simulink model "hnn_3_neurons"  (R2024b)
settings: Solver=VariableStepAuto  StartTime=0.0  StopTime=10.0  RelTol=1e-3
settings Model: Creator=merlin  LastModifiedBy=merlin

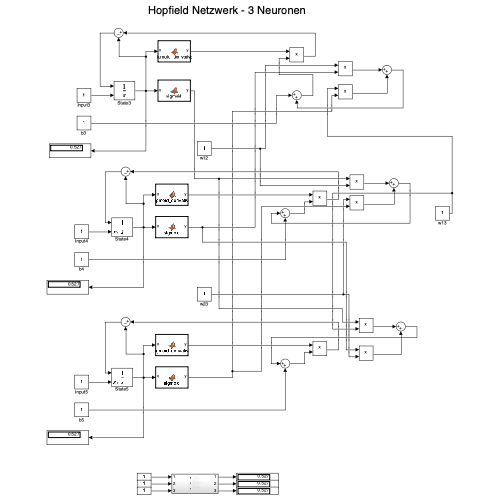
[thumbnail: Simulink's stored preview of the top-level diagram]
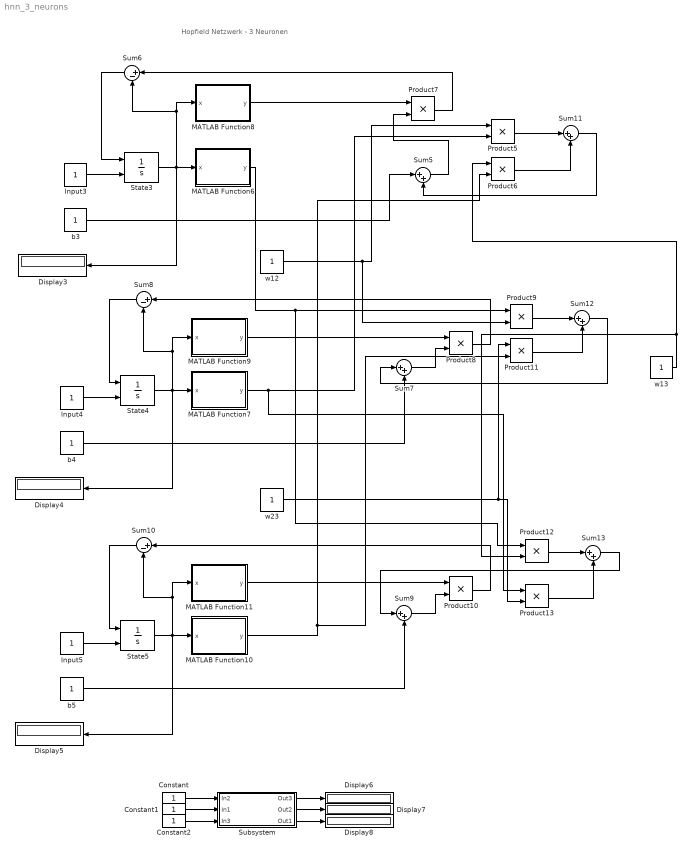
== system hnn_3_neurons ==
  note: Hopfield Netzwerk - 3 Neuronen
  Constant : Constant
  Constant1 : Constant
  Constant2 : Constant
  Display{3..8} (6 alike) : Display
  Input3 : Constant
  Input4 : Constant
  Input5 : Constant
  MATLAB Function10 : MATLAB Function  TreatAsAtomicUnit=on
  MATLAB Function11 : MATLAB Function  TreatAsAtomicUnit=on
  MATLAB Function6 : MATLAB Function  TreatAsAtomicUnit=on
  MATLAB Function7 : MATLAB Function  TreatAsAtomicUnit=on
  MATLAB Function8 : MATLAB Function  TreatAsAtomicUnit=on
  MATLAB Function9 : MATLAB Function  TreatAsAtomicUnit=on
  Product{5..13} (9 alike) : Product
  State3 : Integrator  InitialConditionSource=external
  State4 : Integrator  InitialConditionSource=external
  State5 : Integrator  InitialConditionSource=external
  Subsystem : Subsystem
  Sum10 : Sum  Inputs=|+-
  Sum{5,7,9,11..13} (6 alike) : Sum  Inputs=|++
  Sum6 : Sum  Inputs=|+-
  Sum8 : Sum  Inputs=|+-
  b3 : Constant
  b4 : Constant
  b5 : Constant
  w12 : Constant
  w13 : Constant
  w23 : Constant
  wires:
  w12/1 -> Product9/2, Product5/1
  MATLAB Function7/1(y) -> Product13/1, Product5/2
  Product8/1 -> Sum8/1
  State5/1 -> Display5/1, Sum10/2, MATLAB Function11/1(x), MATLAB Function10/1(x)
  Subsystem/3(Out1) -> Display8/1
  Product7/1 -> Sum6/1
  b3/1 -> Sum5/1
  Input3/1 -> State3/2
  Sum13/1 -> Sum9/1
  Product10/1 -> Sum10/1
  Product13/1 -> Sum13/2
  Subsystem/1(Out3) -> Display6/1
  Sum11/1 -> Sum5/2
  Product6/1 -> Sum11/2
  Input4/1 -> State4/2
  Sum6/1 -> State3/1
  Sum9/1 -> Product10/2
  Sum10/1 -> State5/1
  MATLAB Function8/1(y) -> Product7/1
  w13/1 -> Product12/2, Product6/1
  State4/1 -> Display4/1, Sum8/2, MATLAB Function9/1(x), MATLAB Function7/1(x)
  Constant2/1 -> Subsystem/3(In3)
  b5/1 -> Sum9/2
  Product9/1 -> Sum12/1
  MATLAB Function11/1(y) -> Product10/1
  Subsystem/2(Out2) -> Display7/1
  Sum5/1 -> Product7/2
  Product11/1 -> Sum12/2
  Sum12/1 -> Sum7/1
  Input5/1 -> State5/2
  Product5/1 -> Sum11/1
  Product12/1 -> Sum13/1
  Constant1/1 -> Subsystem/2(In1)
  MATLAB Function10/1(y) -> Product11/2, Product6/2
  b4/1 -> Sum7/2
  State3/1 -> Display3/1, Sum6/2, MATLAB Function8/1(x), MATLAB Function6/1(x)
  MATLAB Function9/1(y) -> Product8/1
  Sum8/1 -> State4/1
  Sum7/1 -> Product8/2
  MATLAB Function6/1(y) -> Product12/1, Product9/1
  Constant/1 -> Subsystem/1(In2)
  w23/1 -> Product13/2, Product11/1

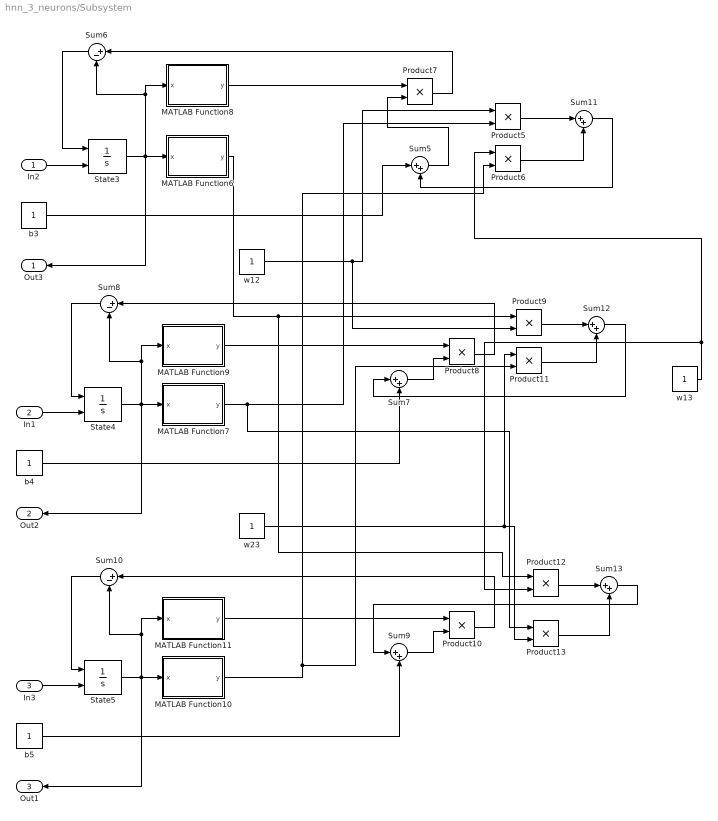
== system hnn_3_neurons/Subsystem ==
  In2 : Inport
  In1 : Inport  Port=2
  In3 : Inport  Port=3
  MATLAB Function10 : MATLAB Function  TreatAsAtomicUnit=on
  MATLAB Function11 : MATLAB Function  TreatAsAtomicUnit=on
  MATLAB Function6 : MATLAB Function  TreatAsAtomicUnit=on
  MATLAB Function7 : MATLAB Function  TreatAsAtomicUnit=on
  MATLAB Function8 : MATLAB Function  TreatAsAtomicUnit=on
  MATLAB Function9 : MATLAB Function  TreatAsAtomicUnit=on
  Product{5..13} (9 alike) : Product
  State3 : Integrator  InitialConditionSource=external
  State4 : Integrator  InitialConditionSource=external
  State5 : Integrator  InitialConditionSource=external
  Sum10 : Sum  Inputs=|+-
  Sum{5,7,9,11..13} (6 alike) : Sum  Inputs=|++
  Sum6 : Sum  Inputs=|+-
  Sum8 : Sum  Inputs=|+-
  b3 : Constant
  b4 : Constant
  b5 : Constant
  w12 : Constant
  w13 : Constant
  w23 : Constant
  Out3 : Outport
  Out2 : Outport  Port=2
  Out1 : Outport  Port=3
  wires:
  Product9/1 -> Sum12/1
  b5/1 -> Sum9/2
  Product13/1 -> Sum13/2
  Sum5/1 -> Product7/2
  b4/1 -> Sum7/2
  Sum10/1 -> State5/1
  MATLAB Function7/1(y) -> Product13/1, Product5/2
  MATLAB Function9/1(y) -> Product8/1
  Product5/1 -> Sum11/1
  w12/1 -> Product9/2, Product5/1
  Sum13/1 -> Sum9/1
  State5/1 -> Out1/1, Sum10/2, MATLAB Function11/1(x), MATLAB Function10/1(x)
  MATLAB Function8/1(y) -> Product7/1
  MATLAB Function11/1(y) -> Product10/1
  Sum9/1 -> Product10/2
  MATLAB Function6/1(y) -> Product12/1, Product9/1
  Product12/1 -> Sum13/1
  MATLAB Function10/1(y) -> Product11/2, Product6/2
  State4/1 -> Out2/1, Sum8/2, MATLAB Function9/1(x), MATLAB Function7/1(x)
  Sum8/1 -> State4/1
  Product8/1 -> Sum8/1
  State3/1 -> Out3/1, Sum6/2, MATLAB Function8/1(x), MATLAB Function6/1(x)
  Sum6/1 -> State3/1
  Product7/1 -> Sum6/1
  b3/1 -> Sum5/1
  Product6/1 -> Sum11/2
  In1/1 -> State4/2
  Sum7/1 -> Product8/2
  In3/1 -> State5/2
  w23/1 -> Product13/2, Product11/1
  Product11/1 -> Sum12/2
  Sum12/1 -> Sum7/1
  Sum11/1 -> Sum5/2
  Product10/1 -> Sum10/1
  w13/1 -> Product12/2, Product6/1
  In2/1 -> State3/2

== matlab function hnn_3_neurons/MATLAB Function7 ==
  data: x input; y output
function y = sigmoid(x)
y = 1 ./ (1 + exp(-x));
end

== matlab function hnn_3_neurons/MATLAB Function8 ==
  data: x input; y output
function y = sigmoid_derivative(x)
sigmoid = 1 ./ (1 + exp(-x));
y = sigmoid .* (1 - sigmoid);
end

== matlab function hnn_3_neurons/MATLAB Function9 ==
  data: x input; y output
function y = sigmoid_derivative(x)
sigmoid = 1 ./ (1 + exp(-x));
y = sigmoid .* (1 - sigmoid);
end

== matlab function hnn_3_neurons/MATLAB Function10 ==
  data: x input; y output
function y = sigmoid(x)
y = 1 ./ (1 + exp(-x));
end

== matlab function hnn_3_neurons/MATLAB Function11 ==
  data: x input; y output
function y = sigmoid_derivative(x)
sigmoid = 1 ./ (1 + exp(-x));
y = sigmoid .* (1 - sigmoid);
end

== matlab function hnn_3_neurons/Subsystem/MATLAB Function10 ==
  data: x input; y output
function y = sigmoid(x)
y = 1 ./ (1 + exp(-x));
end

== matlab function hnn_3_neurons/Subsystem/MATLAB Function11 ==
  data: x input; y output
function y = sigmoid_derivative(x)
sigmoid = 1 ./ (1 + exp(-x));
y = sigmoid .* (1 - sigmoid);
end

== matlab function hnn_3_neurons/Subsystem/MATLAB Function6 ==
  data: x input; y output
function y = sigmoid(x)
y = 1 ./ (1 + exp(-x));
end

== matlab function hnn_3_neurons/MATLAB Function6 ==
  data: x input; y output
function y = sigmoid(x)
y = 1 ./ (1 + exp(-x));
end

== matlab function hnn_3_neurons/Subsystem/MATLAB Function7 ==
  data: x input; y output
function y = sigmoid(x)
y = 1 ./ (1 + exp(-x));
end

== matlab function hnn_3_neurons/Subsystem/MATLAB Function8 ==
  data: x input; y output
function y = sigmoid_derivative(x)
sigmoid = 1 ./ (1 + exp(-x));
y = sigmoid .* (1 - sigmoid);
end

== matlab function hnn_3_neurons/Subsystem/MATLAB Function9 ==
  data: x input; y output
function y = sigmoid_derivative(x)
sigmoid = 1 ./ (1 + exp(-x));
y = sigmoid .* (1 - sigmoid);
end
